simulink model "pll_linear"  (R2022a)
settings: Solver=VariableStepAuto  StartTime=0.0  StopTime=10  RelTol=1e-3
libraries: spsFirstOrderFilterLib x1
settings Model: Creator=fiendchain  LastModifiedBy=fiendchain

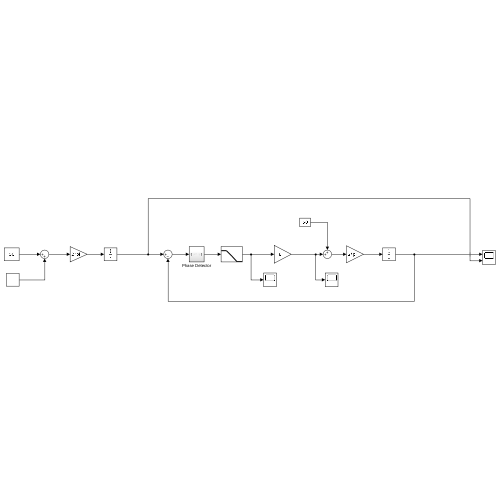
[thumbnail: Simulink's stored preview of the top-level diagram]
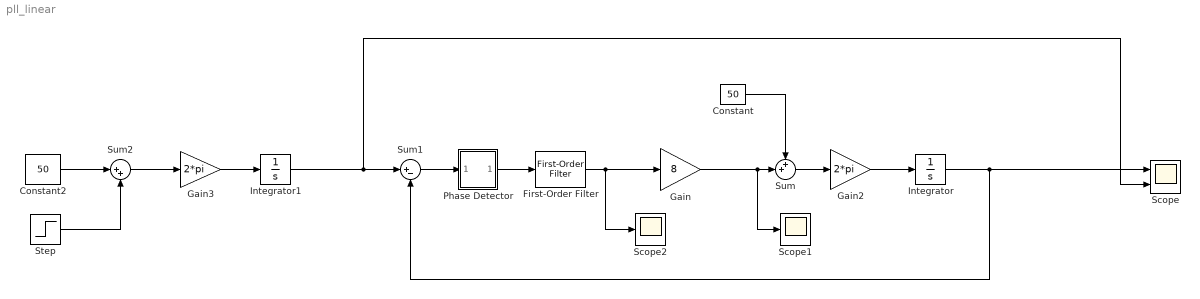
== system pll_linear ==
  Constant : Constant  Value=50
  Constant2 : Constant  Value=50
  First-Order Filter : spsFirstOrderFilterLib/First-Order Filter  FilterType=Lowpass  Tc=1/30  Ts=0  Initialize=on  Vac_Init=[0, 0, 60]  Vdc_Init=0  PlotResponse=off  FreqRange="[0,  200,  1]"
  Gain : Gain  Gain=8
  Gain2 : Gain  Gain=2*pi
  Gain3 : Gain  Gain=2*pi
  Integrator : Integrator
  Integrator1 : Integrator
  Phase Detector : Subsystem
  Scope : Scope  NumInputPorts=2
  Scope1 : Scope
  Scope2 : Scope
  Step : Step  After=-2  SampleTime=0
  Sum : Sum  Inputs=++|
  Sum1 : Sum  Inputs=|+-
  Sum2 : Sum  Inputs=|++
  wires:
  Constant/1 -> Sum/1
  Sum/1 -> Gain2/1
  Sum2/1 -> Gain3/1
  Integrator1/1 -> Scope/2, Sum1/1
  Integrator/1 -> Scope/1, Sum1/2
  Gain2/1 -> Integrator/1
  Sum1/1 -> Phase Detector/1(In1)
  Phase Detector/1(Out1) -> First-Order Filter/1
  Gain3/1 -> Integrator1/1
  Constant2/1 -> Sum2/1
  Step/1 -> Sum2/2
  First-Order Filter/1 -> Gain/1, Scope2/1
  Gain/1 -> Scope1/1, Sum/2

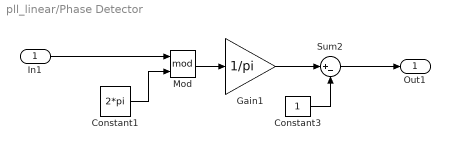
== system pll_linear/Phase Detector ==
  In1 : Inport
  Constant1 : Constant  Value=2*pi
  Constant3 : Constant
  Gain1 : Gain  Gain=1/pi
  Mod : Math  Operator=mod
  Sum2 : Sum  Inputs=|+-
  Out1 : Outport
  wires:
  Constant1/1 -> Mod/2
  Mod/1 -> Gain1/1
  Gain1/1 -> Sum2/1
  Constant3/1 -> Sum2/2
  In1/1 -> Mod/1
  Sum2/1 -> Out1/1
